simulink model "Doppelpendel_EKF_2016a"  (R2016a)
settings: Solver=ode45  StartTime=0.0  StopTime=10
undefined symbols (not defined in the file or in its folder): parDP, parEKF, parLQR
libraries: cstblocks x3
(part 1 of 2)
settings Model: Creator=tg  LastModifiedBy=Meiner
settings DataIOCC: LimitDataPoints=on  SaveFormat=Array  SignalLoggingSaveFormat=ModelDataLogs
settings OptimizationCC: ExpressionDepthLimit=2147483647  InitFltsAndDblsToZero=on
settings DebuggingCC: UnderspecifiedInitializationDetection=Classic  MergeDetectMultiDrivingBlocksExec=none  SolverPrmCheckMsg=warning  FcnCallInpInsideContextMsg=EnableAllAsWarning  StateNameClashWarn=warning
settings HardwareCC: ProdBitPerPointer=32  ProdLargestAtomicFloat=None  ProdIntDivRoundTo=Undefined  ProdEndianess=Unspecified  ProdWordSize=32  ProdHWDeviceType=32-bit Generic
settings ModelReferenceCC: PropagateSignalLabelsOutOfModel=off
settings SFSimCC: SimParseCustomCode=off
settings GRTTargetCC: CombineOutputUpdateFcns=off  GRTInterface=on

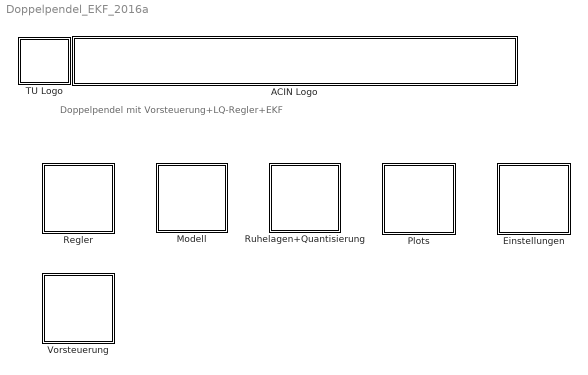
== system Doppelpendel_EKF_2016a ==
  note: Doppelpendel mit Vorsteuerung+LQ-Regler+EKF
  ACIN Logo : Subsystem
      mask init:
      | s = get_param(gcb,'UserData');
      mask Display:
      | image(s.logo,[0 0 439 45]);
      | %axis image
  Einstellungen : Subsystem
  Modell : Subsystem
  Plots : Subsystem
  Regler : Subsystem
  Ruhelagen+Quantisierung : Subsystem
  TU Logo : Subsystem
      mask init:
      | s = get_param(gcb,'UserData');
      mask Display: image(s.logo,[0 0 45 45]);
  Vorsteuerung : Subsystem

== system Doppelpendel_EKF_2016a/ACIN Logo ==

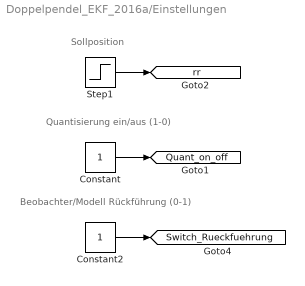
== system Doppelpendel_EKF_2016a/Einstellungen ==
  note: Sollposition
  note: Quantisierung ein/aus (1-0)
  note: Beobachter/Modell Rückführung (0-1)
  Constant : Constant
  Constant2 : Constant
  Step1 : Step  After=0.1  SampleTime=parLQR.Ta
  tag scope: Quant_on_off=global, Switch_Rueckfuehrung=global, rr=global
  wires:
  Step1/1 -> [rr]
  Constant/1 -> [Quant_on_off]
  Constant2/1 -> [Switch_Rueckfuehrung]

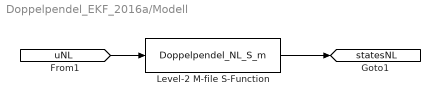
== system Doppelpendel_EKF_2016a/Modell ==
  Level-2 M-file S-Function : M-S-Function  FunctionName=Doppelpendel_NL_S_m  Parameters=parDP.phi10,parDP.omega10,parDP.phi20,parDP.omega20,parDP.s0,parDP.w0,parDP.l1,parDP.l2,parDP.a1,parDP.a2,parDP.m1,parDP.m2,parDP.J1,parDP.J2,parDP.d1,parDP.d2
  tag scope: statesNL=global
  wires:
  Level-2 M-file S-Function/1 -> [statesNL]
  [uNL] -> Level-2 M-file S-Function/1

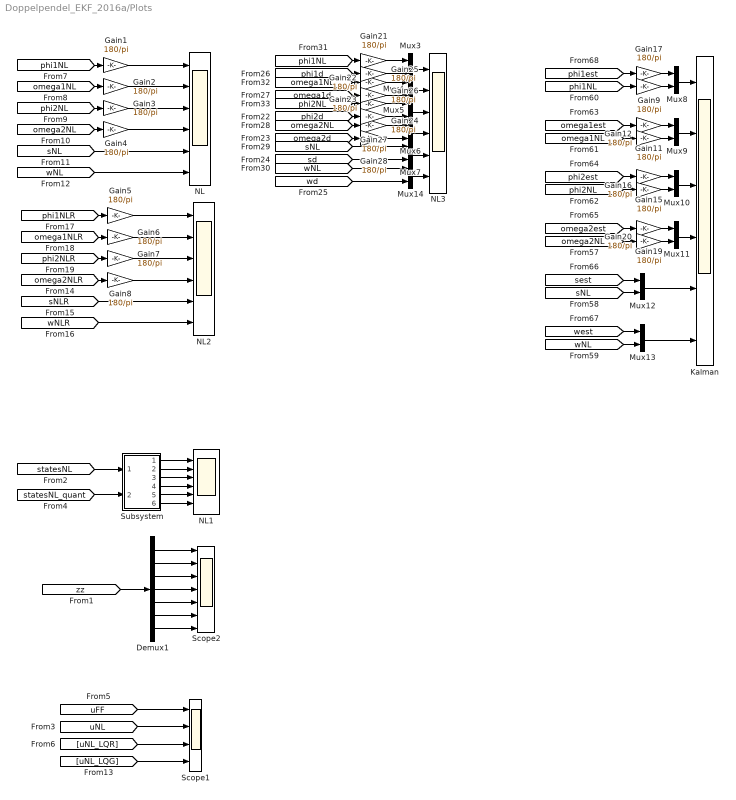
== system Doppelpendel_EKF_2016a/Plots ==
  Demux1 : Demux  Outputs=7
  Gain{1..9,11..12,15..17,19..28} (24 alike) : Gain  Gain=180/pi
  Kalman : Scope  NumInputPorts=6
  Mux{3..14} (12 alike) : Mux  Inputs=2
  NL{,1..3} (4 alike) : Scope  NumInputPorts=6
  Scope1 : Scope  NumInputPorts=4
  Scope2 : Scope  NumInputPorts=7
  Subsystem : Subsystem
  wires:
  [omega1NL] -> Gain2/1
  [omega2NL] -> Gain4/1
  [sNL] -> NL/5
  [wNL] -> NL/6
  Gain1/1 -> NL/1
  Gain2/1 -> NL/2
  Gain3/1 -> NL/3
  Gain4/1 -> NL/4
  [phi1NL] -> Gain1/1
  [phi2NL] -> Gain3/1
  [statesNL] -> Subsystem/1(In1)
  [statesNL_quant] -> Subsystem/2(In2)
  Subsystem/1(Out1) -> NL1/1
  Subsystem/2(Out2) -> NL1/2
  Subsystem/3(Out3) -> NL1/3
  Subsystem/4(Out4) -> NL1/4
  Subsystem/5(Out5) -> NL1/5
  Subsystem/6(Out6) -> NL1/6
  [omega1NL] -> Gain22/1
  [omega2NL] -> Gain24/1
  [phi1NL] -> Gain21/1
  [phi2NL] -> Gain23/1
  Mux3/1 -> NL3/1
  Mux4/1 -> NL3/2
  Mux5/1 -> NL3/3
  Mux6/1 -> NL3/4
  Mux7/1 -> NL3/5
  Mux14/1 -> NL3/6
  Gain21/1 -> Mux3/1
  Gain22/1 -> Mux4/1
  Gain23/1 -> Mux5/1
  Gain24/1 -> Mux6/1
  [sNL] -> Mux7/1
  [wNL] -> Mux14/1
  [phi1d] -> Gain25/1
  [omega1d] -> Gain26/1
  [phi2d] -> Gain27/1
  [omega2d] -> Gain28/1
  Gain25/1 -> Mux3/2
  Gain26/1 -> Mux4/2
  Gain27/1 -> Mux5/2
  Gain28/1 -> Mux6/2
  [sd] -> Mux7/2
  [wd] -> Mux14/2
  Demux1/1 -> Scope2/1
  Demux1/2 -> Scope2/2
  Demux1/3 -> Scope2/3
  Demux1/4 -> Scope2/4
  Demux1/5 -> Scope2/5
  Demux1/6 -> Scope2/6
  Demux1/7 -> Scope2/7
  [zz] -> Demux1/1
  Mux13/1 -> Kalman/6
  Mux12/1 -> Kalman/5
  Mux11/1 -> Kalman/4
  [omega1NL] -> Gain12/1
  [omega2NL] -> Gain20/1
  [phi1NL] -> Gain9/1
  [phi2NL] -> Gain16/1
  [sest] -> Mux12/1
  [west] -> Mux13/1
  [sNL] -> Mux12/2
  [wNL] -> Mux13/2
  Gain9/1 -> Mux8/2
  Gain17/1 -> Mux8/1
  [phi1est] -> Gain17/1
  Mux8/1 -> Kalman/1
  Gain12/1 -> Mux9/2
  Gain11/1 -> Mux9/1
  Mux9/1 -> Kalman/2
  [omega1est] -> Gain11/1
  Gain16/1 -> Mux10/2
  Gain15/1 -> Mux10/1
  [phi2est] -> Gain15/1
  Mux10/1 -> Kalman/3
  Gain20/1 -> Mux11/2
  Gain19/1 -> Mux11/1
  [omega2est] -> Gain19/1
  [uFF] -> Scope1/1
  [uNL] -> Scope1/2
  [uNL_LQR] -> Scope1/3
  [uNL_LQG] -> Scope1/4
  [omega1NLR] -> Gain6/1
  [omega2NLR] -> Gain8/1
  [sNLR] -> NL2/5
  [wNLR] -> NL2/6
  Gain5/1 -> NL2/1
  Gain6/1 -> NL2/2
  Gain7/1 -> NL2/3
  Gain8/1 -> NL2/4
  [phi1NLR] -> Gain5/1
  [phi2NLR] -> Gain7/1

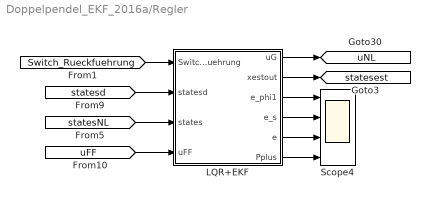
== system Doppelpendel_EKF_2016a/Regler ==
  LQR+EKF : MATLAB Function  TreatAsAtomicUnit=on
      settings: PermitHierarchicalResolution=ParametersOnly
  Scope4 : Scope  NumInputPorts=4
  tag scope: statesest=global, uNL=global
  wires:
  LQR+EKF/3(e_phi1) -> Scope4/1
  LQR+EKF/4(e_s) -> Scope4/2
  LQR+EKF/5(e) -> Scope4/3
  LQR+EKF/2(xestout) -> [statesest]
  [statesd] -> LQR+EKF/2(statesd)
  [uFF] -> LQR+EKF/4(uFF)
  [statesNL] -> LQR+EKF/3(states)
  LQR+EKF/6(Pplus) -> Scope4/4
  LQR+EKF/1(uG) -> [uNL]
  [Switch_Rueckfuehrung] -> LQR+EKF/1(Switch_Rueckfuehrung)

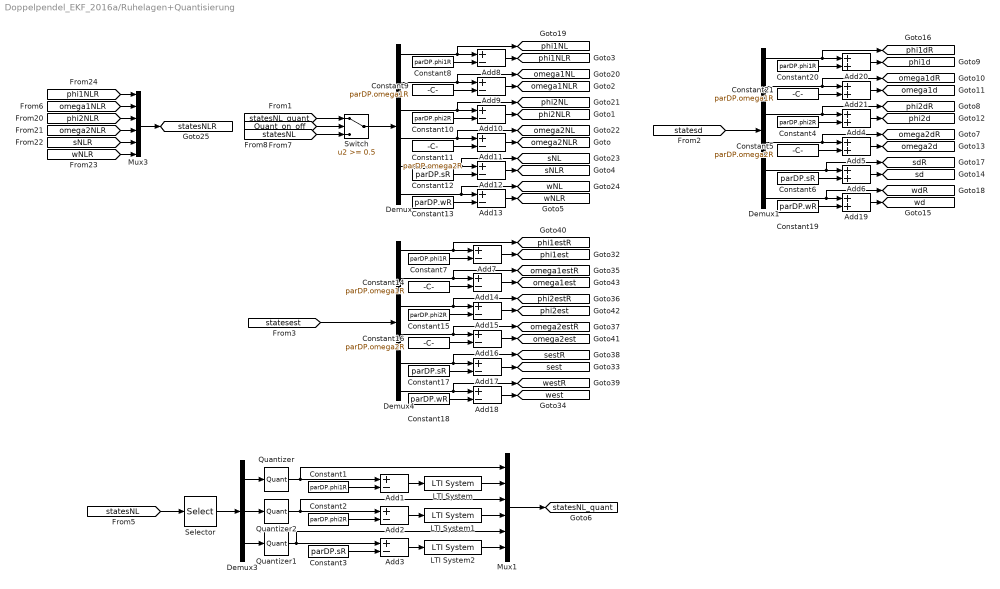
== system Doppelpendel_EKF_2016a/Ruhelagen+Quantisierung ==
  Add{1..3,7..18} (15 alike) : Sum  Inputs=+-
  Add{4..6,19..21} (6 alike) : Sum
  Constant{1,7..8,20} (4 alike) : Constant  Value=parDP.phi1R
  Constant{2,4,10,15} (4 alike) : Constant  Value=parDP.phi2R
  Constant11 : Constant  Value=parDP.omega2R
  Constant{3,6,12,17} (4 alike) : Constant  Value=parDP.sR
  Constant13 : Constant  Value=parDP.wR
  Constant14 : Constant  Value=parDP.omega1R
  Constant16 : Constant  Value=parDP.omega2R
  Constant18 : Constant  Value=parDP.wR
  Constant19 : Constant  Value=parDP.wR
  Constant21 : Constant  Value=parDP.omega1R
  Constant5 : Constant  Value=parDP.omega2R
  Constant9 : Constant  Value=parDP.omega1R
  Demux : Demux  Outputs=6
  Demux1 : Demux  Outputs=6
  Demux3 : Demux  Outputs=3
  Demux4 : Demux  Outputs=6
  LTI System : cstblocks/LTI System  sys=Fd_diff  IC=[]
  LTI System1 : cstblocks/LTI System  sys=Fd_diff  IC=[]
  LTI System2 : cstblocks/LTI System  sys=Fd_diff  IC=[]
  Mux1 : Mux  Inputs=6
  Mux3 : Mux  Inputs=6
  Quantizer : Quantizer  QuantizationInterval=Phiquantisierung  SampleTime=parLQR.Ta
  Quantizer1 : Quantizer  QuantizationInterval=Wegquantisierung  SampleTime=parLQR.Ta
  Quantizer2 : Quantizer  QuantizationInterval=Phiquantisierung  SampleTime=parLQR.Ta
  Selector : Selector  InputPortWidth=6  IndexOptions=Index vector (dialog)  Indices=[1 3 5]  OutputSizes=1
  Switch : Switch  Threshold=0.5
  tag scope: omega1NL=global, omega1NLR=global, omega1d=global, omega1dR=global, omega1est=global, omega1estR=global, omega2NL=global, omega2NLR=global, omega2d=global, omega2dR=global, omega2est=global, omega2estR=global, phi1NL=global, phi1NLR=global, phi1d=global, phi1dR=global, phi1est=global, phi1estR=global, phi2NL=global, phi2NLR=global, phi2d=global, phi2dR=global, phi2est=global, phi2estR=global, sNL=global, sNLR=global, sd=global, sdR=global, sest=global, sestR=global, statesNLR=global, statesNL_quant=global, wNL=global, wNLR=global, wd=global, wdR=global, west=global, westR=global
  wires:
  [phi1NLR] -> Mux3/1
  [omega1NLR] -> Mux3/2
  [phi2NLR] -> Mux3/3
  [omega2NLR] -> Mux3/4
  [sNLR] -> Mux3/5
  [wNLR] -> Mux3/6
  Mux3/1 -> [statesNLR]
  Demux/1 -> Add8/1, [phi1NL]
  Demux/2 -> Add9/1, [omega1NL]
  Demux/3 -> Add10/1, [phi2NL]
  Demux/4 -> Add11/1, [omega2NL]
  Demux/5 -> Add12/1, [sNL]
  Demux/6 -> Add13/1, [wNL]
  Constant8/1 -> Add8/2
  Constant9/1 -> Add9/2
  Constant10/1 -> Add10/2
  Constant11/1 -> Add11/2
  Constant12/1 -> Add12/2
  Constant13/1 -> Add13/2
  Add8/1 -> [phi1NLR]
  Add9/1 -> [omega1NLR]
  Add10/1 -> [phi2NLR]
  Add11/1 -> [omega2NLR]
  Add12/1 -> [sNLR]
  Add13/1 -> [wNLR]
  Constant7/1 -> Add7/2
  Constant14/1 -> Add14/2
  Constant15/1 -> Add15/2
  Constant16/1 -> Add16/2
  Constant17/1 -> Add17/2
  Constant18/1 -> Add18/2
  Demux4/1 -> Add7/1, [phi1estR]
  Add7/1 -> [phi1est]
  Demux4/2 -> [omega1estR], Add14/1
  Add14/1 -> [omega1est]
  Demux4/3 -> [phi2estR], Add15/1
  Add15/1 -> [phi2est]
  Demux4/4 -> [omega2estR], Add16/1
  Add16/1 -> [omega2est]
  Demux4/5 -> [sestR], Add17/1
  Add17/1 -> [sest]
  Demux4/6 -> [westR], Add18/1
  Add18/1 -> [west]
  [statesest] -> Demux4/1
  [statesNL] -> Selector/1
  Selector/1 -> Demux3/1
  Demux3/2 -> Quantizer2/1
  Demux3/1 -> Quantizer/1
  Demux3/3 -> Quantizer1/1
  Mux1/1 -> [statesNL_quant]
  LTI System/1 -> Mux1/2
  LTI System2/1 -> Mux1/6
  Switch/1 -> Demux/1
  [Quant_on_off] -> Switch/2
  [statesNL_quant] -> Switch/1
  [statesNL] -> Switch/3
  LTI System1/1 -> Mux1/4
  Add1/1 -> LTI System/1
  Add2/1 -> LTI System1/1
  Add3/1 -> LTI System2/1
  Constant1/1 -> Add1/2
  Constant2/1 -> Add2/2
  Constant3/1 -> Add3/2
  Quantizer1/1 -> Add3/1, Mux1/5
  Quantizer2/1 -> Add2/1, Mux1/3
  Quantizer/1 -> Add1/1, Mux1/1
  Demux1/1 -> Add20/1, [phi1dR]
  Demux1/2 -> Add21/1, [omega1dR]
  Demux1/3 -> Add4/1, [phi2dR]
  Demux1/4 -> Add5/1, [omega2dR]
  Demux1/5 -> Add6/1, [sdR]
  Demux1/6 -> Add19/1, [wdR]
  Constant5/1 -> Add5/2
  Constant6/1 -> Add6/2
  Constant19/1 -> Add19/2
  Add20/1 -> [phi1d]
  Add21/1 -> [omega1d]
  Add4/1 -> [phi2d]
  Add5/1 -> [omega2d]
  Add6/1 -> [sd]
  Add19/1 -> [wd]
  [statesd] -> Demux1/1
  Constant21/1 -> Add21/2
  Constant20/1 -> Add20/2
  Constant4/1 -> Add4/2

== system Doppelpendel_EKF_2016a/TU Logo ==

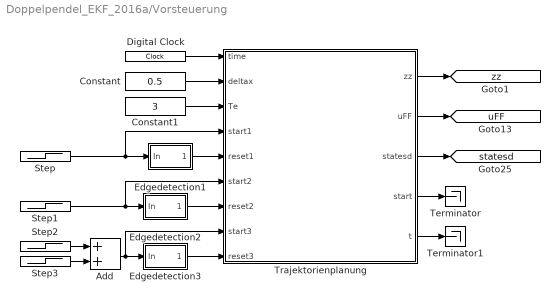
== system Doppelpendel_EKF_2016a/Vorsteuerung ==
  Add : Sum
  Constant : Constant  Value=0.5
  Constant1 : Constant  Value=3
  Digital Clock : DigitalClock  SampleTime=parLQR.Ta
  Edgedetection1 : Subsystem
  Edgedetection2 : Subsystem
  Edgedetection3 : Subsystem
  Step : Step  Time=2  SampleTime=0
  Step1 : Step  Time=6  SampleTime=0
  Step2 : Step  Time=14  After=-1  SampleTime=0
  Step3 : Step  Time=10  SampleTime=0
  Terminator : Terminator
  Terminator1 : Terminator
  Trajektorienplanung : MATLAB Function  TreatAsAtomicUnit=on
      settings: PermitHierarchicalResolution=ParametersOnly
  tag scope: statesd=global, uFF=global, zz=global
  wires:
  Trajektorienplanung/1(zz) -> [zz]
  Trajektorienplanung/5(t) -> Terminator1/1
  Trajektorienplanung/4(start) -> Terminator/1
  Step3/1 -> Add/2
  Step2/1 -> Add/1
  Edgedetection3/1(Out1) -> Trajektorienplanung/9(reset3)
  Step1/1 -> Edgedetection2/1(In), Trajektorienplanung/6(start2)
  Edgedetection2/1(Out1) -> Trajektorienplanung/7(reset2)
  Edgedetection1/1(Out1) -> Trajektorienplanung/5(reset1)
  Digital Clock/1 -> Trajektorienplanung/1(time)
  Trajektorienplanung/3(statesd) -> [statesd]
  Step/1 -> Edgedetection1/1(In), Trajektorienplanung/4(start1)
  Trajektorienplanung/2(uFF) -> [uFF]
  Constant/1 -> Trajektorienplanung/2(deltax)
  Constant1/1 -> Trajektorienplanung/3(Te)
  Add/1 -> Edgedetection3/1(In), Trajektorienplanung/8(start3)

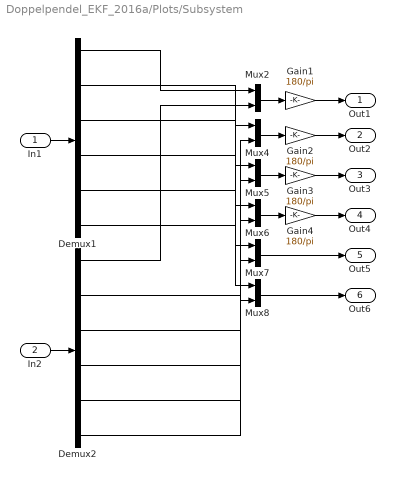
== system Doppelpendel_EKF_2016a/Plots/Subsystem ==
  In1 : Inport
  In2 : Inport  Port=2
  Demux1 : Demux  Outputs=6
  Demux2 : Demux  Outputs=6
  Gain{1..4} (4 alike) : Gain  Gain=180/pi
  Mux{2,4..8} (6 alike) : Mux  Inputs=2
  Out1 : Outport
  Out2 : Outport  Port=2
  Out3 : Outport  Port=3
  Out4 : Outport  Port=4
  Out5 : Outport  Port=5
  Out6 : Outport  Port=6
  wires:
  Demux1/1 -> Mux2/1
  Demux2/1 -> Mux2/2
  Demux2/2 -> Mux4/2
  Demux2/3 -> Mux5/2
  Demux2/4 -> Mux6/2
  Demux2/5 -> Mux7/2
  Demux2/6 -> Mux8/2
  Demux1/6 -> Mux8/1
  Demux1/5 -> Mux7/1
  Demux1/2 -> Mux4/1
  Demux1/3 -> Mux5/1
  Demux1/4 -> Mux6/1
  Mux2/1 -> Gain1/1
  Mux4/1 -> Gain2/1
  In1/1 -> Demux1/1
  Mux5/1 -> Gain3/1
  Mux6/1 -> Gain4/1
  Mux7/1 -> Out5/1
  Mux8/1 -> Out6/1
  In2/1 -> Demux2/1
  Gain1/1 -> Out1/1
  Gain2/1 -> Out2/1
  Gain3/1 -> Out3/1
  Gain4/1 -> Out4/1

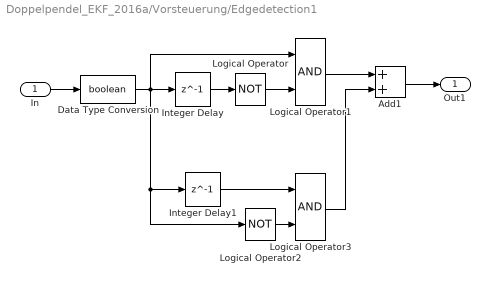
== system Doppelpendel_EKF_2016a/Vorsteuerung/Edgedetection1 ==
  In : Inport
  Add1 : Sum
  Data Type Conversion : DataTypeConversion  OutDataTypeStr=boolean  SaturateOnIntegerOverflow=on  RndMeth=Zero
  Integer Delay : Delay  DelayLength=1  InputProcessing=Inherited  SampleTime=parLQR.Ta
  Integer Delay1 : Delay  DelayLength=1  InputProcessing=Inherited  SampleTime=parLQR.Ta
  Logical Operator : Logic  Operator=NOT  Inputs=1
  Logical Operator1 : Logic
  Logical Operator2 : Logic  Operator=NOT  Inputs=1
  Logical Operator3 : Logic
  Out1 : Outport
  wires:
  In/1 -> Data Type Conversion/1
  Integer Delay/1 -> Logical Operator/1
  Data Type Conversion/1 -> Logical Operator1/1, Integer Delay/1, Integer Delay1/1, Logical Operator2/1
  Logical Operator/1 -> Logical Operator1/2
  Logical Operator2/1 -> Logical Operator3/2
  Integer Delay1/1 -> Logical Operator3/1
  Logical Operator1/1 -> Add1/1
  Logical Operator3/1 -> Add1/2
  Add1/1 -> Out1/1

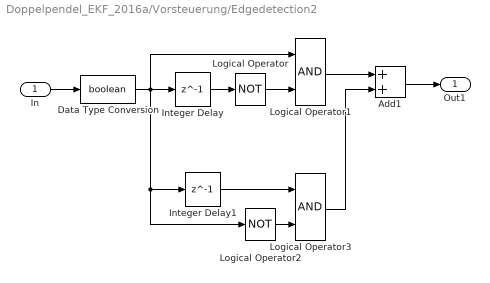
== system Doppelpendel_EKF_2016a/Vorsteuerung/Edgedetection2 ==
  In : Inport
  Add1 : Sum
  Data Type Conversion : DataTypeConversion  OutDataTypeStr=boolean  SaturateOnIntegerOverflow=on  RndMeth=Zero
  Integer Delay : Delay  DelayLength=1  InputProcessing=Inherited  SampleTime=parLQR.Ta
  Integer Delay1 : Delay  DelayLength=1  InputProcessing=Inherited  SampleTime=parLQR.Ta
  Logical Operator : Logic  Operator=NOT  Inputs=1
  Logical Operator1 : Logic
  Logical Operator2 : Logic  Operator=NOT  Inputs=1
  Logical Operator3 : Logic
  Out1 : Outport
  wires:
  Add1/1 -> Out1/1
  Logical Operator3/1 -> Add1/2
  Logical Operator1/1 -> Add1/1
  Integer Delay1/1 -> Logical Operator3/1
  Logical Operator2/1 -> Logical Operator3/2
  Logical Operator/1 -> Logical Operator1/2
  Data Type Conversion/1 -> Logical Operator2/1, Integer Delay1/1, Integer Delay/1, Logical Operator1/1
  Integer Delay/1 -> Logical Operator/1
  In/1 -> Data Type Conversion/1

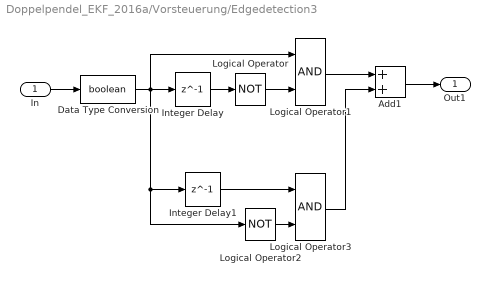
== system Doppelpendel_EKF_2016a/Vorsteuerung/Edgedetection3 ==
  In : Inport
  Add1 : Sum
  Data Type Conversion : DataTypeConversion  OutDataTypeStr=boolean  SaturateOnIntegerOverflow=on  RndMeth=Zero
  Integer Delay : Delay  DelayLength=1  InputProcessing=Inherited  SampleTime=parLQR.Ta
  Integer Delay1 : Delay  DelayLength=1  InputProcessing=Inherited  SampleTime=parLQR.Ta
  Logical Operator : Logic  Operator=NOT  Inputs=1
  Logical Operator1 : Logic
  Logical Operator2 : Logic  Operator=NOT  Inputs=1
  Logical Operator3 : Logic
  Out1 : Outport
  wires:
  In/1 -> Data Type Conversion/1
  Integer Delay/1 -> Logical Operator/1
  Data Type Conversion/1 -> Logical Operator1/1, Integer Delay/1, Integer Delay1/1, Logical Operator2/1
  Logical Operator/1 -> Logical Operator1/2
  Logical Operator2/1 -> Logical Operator3/2
  Integer Delay1/1 -> Logical Operator3/1
  Logical Operator1/1 -> Add1/1
  Logical Operator3/1 -> Add1/2
  Add1/1 -> Out1/1
